simulink model "Klatt2"  (R2014a)
settings: Solver=ode45  StartTime=0  StopTime=6200  MaxStep=0.1  RelTol=1e-3
libraries: simulink x1
settings Model: Creator=OshoGupta  LastModifiedBy=abc
settings DataIOCC: SignalLoggingSaveFormat=ModelDataLogs
settings OptimizationCC: ExpressionDepthLimit=2147483647
settings DebuggingCC: UnderspecifiedInitializationDetection=Classic  FcnCallInpInsideContextMsg=EnableAllAsWarning  StateNameClashWarn=warning

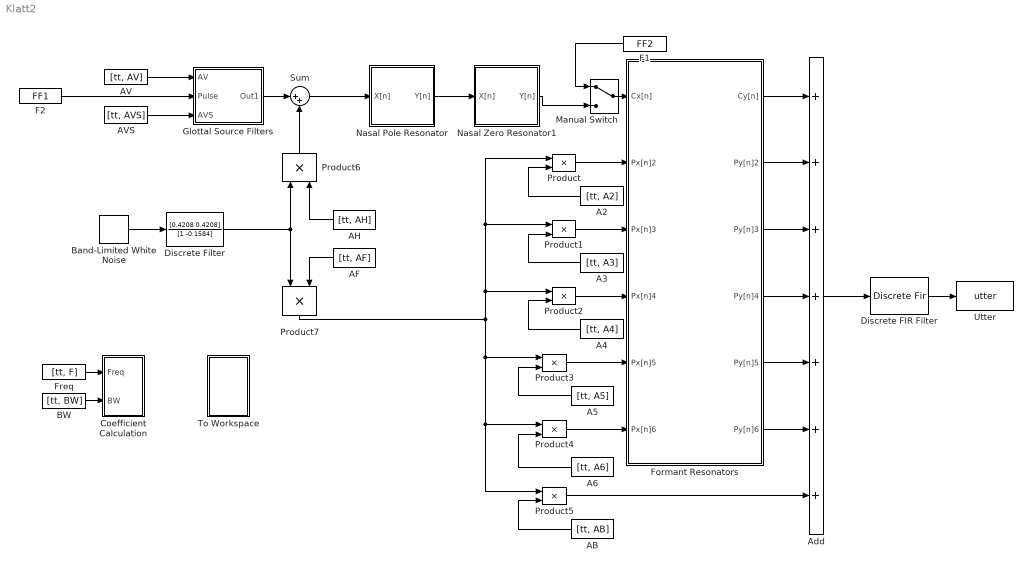
== system Klatt2 ==
  A2 : FromWorkspace  VariableName=[tt, A2]  SampleTime=0
  A3 : FromWorkspace  VariableName=[tt, A3]  SampleTime=0
  A4 : FromWorkspace  VariableName=[tt, A4]  SampleTime=0
  A5 : FromWorkspace  VariableName=[tt, A5]  SampleTime=0
  A6 : FromWorkspace  VariableName=[tt, A6]  SampleTime=0
  AB : FromWorkspace  VariableName=[tt, AB]  SampleTime=0
  AF : FromWorkspace  VariableName=[tt, AF]  SampleTime=0
  AH : FromWorkspace  VariableName=[tt, AH]  SampleTime=0
  AV : FromWorkspace  VariableName=[tt, AV]  SampleTime=0
  AVS : FromWorkspace  VariableName=[tt, AVS]  SampleTime=0
  Add : Sum  Inputs=+++++++
  BW : FromWorkspace  VariableName=[tt, BW]  SampleTime=0
  Band-Limited White Noise : simulink/Sources/Band-Limited White Noise  Cov=[0.1]  Ts=0.1  seed=[23341]
  Coefficient Calculation : Subsystem
  Discrete FIR Filter : DiscreteFir  Coefficients=[1 -0.98]
  Discrete Filter : DiscreteFilter  Numerator=[0.4208 0.4208]  Denominator=[1 -0.1584]
  F1 : FromWorkspace  VariableName=FF2  SampleTime=0
  F2 : FromWorkspace  VariableName=FF1  SampleTime=0
  Formant Resonators : Subsystem
  Freq : FromWorkspace  VariableName=[tt, F]  SampleTime=0
  Glottal Source Filters : Subsystem
  Manual Switch : ManualSwitch
  Nasal Pole Resonator : Subsystem
  Nasal Zero Resonator1 : Subsystem
  Product{,1..7} (8 alike) : Product  RndMeth=Zero
  Sum : Sum  Inputs=|++
  To Workspace : Subsystem
  Utter : ToWorkspace  VariableName=utter  SaveFormat=Timeseries  SampleTime=-1
  wires:
  Freq/1 -> Coefficient Calculation/1(Freq)
  BW/1 -> Coefficient Calculation/2(BW)
  Nasal Pole Resonator/1(Y[n]) -> Nasal Zero Resonator1/1(X[n])
  A2/1 -> Product/2
  Product/1 -> Formant Resonators/2(Px[n]2)
  A3/1 -> Product1/2
  Product1/1 -> Formant Resonators/3(Px[n]3)
  A4/1 -> Product2/2
  Product2/1 -> Formant Resonators/4(Px[n]4)
  A5/1 -> Product3/2
  Product3/1 -> Formant Resonators/5(Px[n]5)
  Product4/1 -> Formant Resonators/6(Px[n]6)
  AB/1 -> Product5/2
  Product7/1 -> Product4/1, Product5/1, Product3/1, Product/1, Product1/1, Product2/1
  Formant Resonators/1(Cy[n]) -> Add/1
  Formant Resonators/2(Py[n]2) -> Add/2
  Formant Resonators/3(Py[n]3) -> Add/3
  Formant Resonators/4(Py[n]4) -> Add/4
  Formant Resonators/5(Py[n]5) -> Add/5
  Formant Resonators/6(Py[n]6) -> Add/6
  Product5/1 -> Add/7
  A6/1 -> Product4/2
  Band-Limited White Noise/1 -> Discrete Filter/1
  Discrete Filter/1 -> Product7/1, Product6/1
  AH/1 -> Product6/2
  AF/1 -> Product7/2
  Sum/1 -> Nasal Pole Resonator/1(X[n])
  Nasal Zero Resonator1/1(Y[n]) -> Manual Switch/2
  F1/1 -> Manual Switch/1
  AVS/1 -> Glottal Source Filters/3(AVS)
  AV/1 -> Glottal Source Filters/1(AV)
  Glottal Source Filters/1(Out1) -> Sum/1
  Add/1 -> Discrete FIR Filter/1
  Discrete FIR Filter/1 -> Utter/1
  F2/1 -> Glottal Source Filters/2(Pulse)
  Manual Switch/1 -> Formant Resonators/1(Cx[n])
  Product6/1 -> Sum/2

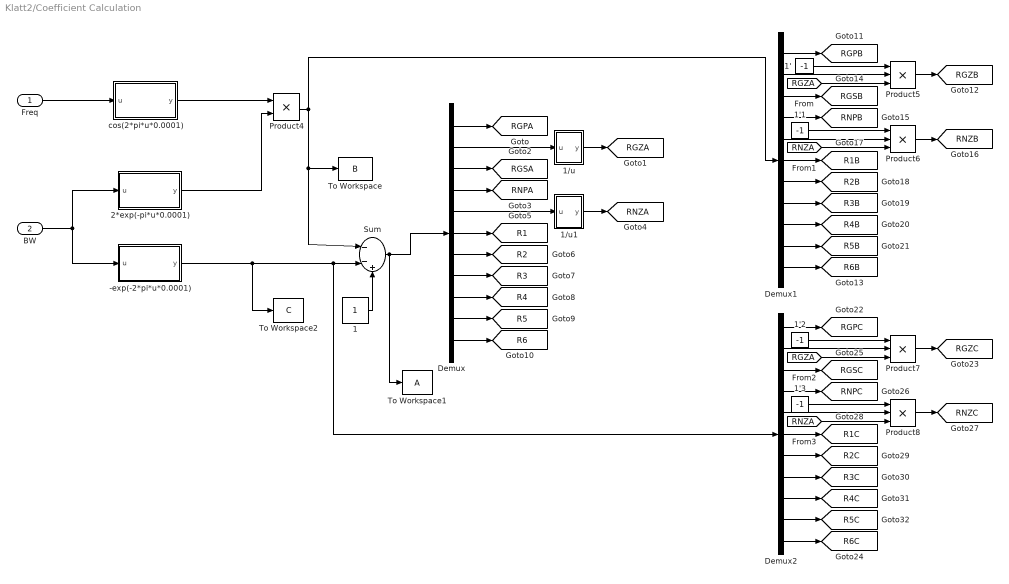
== system Klatt2/Coefficient Calculation ==
  Freq : Inport
  BW : Inport  Port=2
  -exp(-2*pi*u*0.0001) : MATLAB Function  TreatAsAtomicUnit=on
  1 : Constant
  1'{,1..3} (4 alike) : Constant  Value=-1
  1/u : MATLAB Function  TreatAsAtomicUnit=on
  1/u1 : MATLAB Function  TreatAsAtomicUnit=on
  2*exp(-pi*u*0.0001) : MATLAB Function  TreatAsAtomicUnit=on
  Demux : Demux  Outputs=11
  Demux1 : Demux  Outputs=11
  Demux2 : Demux  Outputs=11
  Product4 : Product  RndMeth=Zero
  Product5 : Product  Inputs=3  RndMeth=Zero
  Product6 : Product  Inputs=3  RndMeth=Zero
  Product7 : Product  Inputs=3  RndMeth=Zero
  Product8 : Product  Inputs=***  RndMeth=Zero
  Sum : Sum  Inputs=|--+
  To Workspace : ToWorkspace  VariableName=B  SaveFormat=Timeseries  SampleTime=-1
  To Workspace1 : ToWorkspace  VariableName=A  SaveFormat=Timeseries  SampleTime=-1
  To Workspace2 : ToWorkspace  VariableName=C  SaveFormat=Timeseries  SampleTime=-1
  cos(2*pi*u*0.0001) : MATLAB Function  TreatAsAtomicUnit=on
  tag scope: R1=global, R1B=global, R1C=global, R2=global, R2B=global, R2C=global, R3=global, R3B=global, R3C=global, R4=global, R4B=global, R4C=global, R5=global, R5B=global, R5C=global, R6=global, R6B=global, R6C=global, RGPA=global, RGPB=global, RGPC=global, RGSA=global, RGSB=global, RGSC=global, RGZA=global, RGZB=global, RGZC=global, RNPA=global, RNPB=global, RNPC=global, RNZA=global, RNZB=global, RNZC=global
  wires:
  BW/1 -> 2*exp(-pi*u*0.0001)/1(u), -exp(-2*pi*u*0.0001)/1(u)
  Freq/1 -> cos(2*pi*u*0.0001)/1(u)
  cos(2*pi*u*0.0001)/1(y) -> Product4/1
  2*exp(-pi*u*0.0001)/1(y) -> Product4/2
  Product4/1 -> Demux1/1, To Workspace/1, Sum/1
  -exp(-2*pi*u*0.0001)/1(y) -> To Workspace2/1, Sum/2, Demux2/1
  1/1 -> Sum/3
  Sum/1 -> Demux/1, To Workspace1/1
  Demux/1 -> [RGPA]
  Demux/3 -> [RGSA]
  Demux/4 -> [RNPA]
  Demux/6 -> [R1]
  Demux/7 -> [R2]
  Demux/8 -> [R3]
  Demux/9 -> [R4]
  Demux/10 -> [R5]
  Demux/11 -> [R6]
  Demux/5 -> 1/u1/1(u)
  1/u1/1(y) -> [RNZA]
  Product5/1 -> [RGZB]
  Demux1/2 -> Product5/2
  Demux1/1 -> [RGPB]
  Demux1/3 -> [RGSB]
  Demux1/4 -> [RNPB]
  Demux1/6 -> [R1B]
  Demux1/7 -> [R2B]
  Demux1/8 -> [R3B]
  Demux1/9 -> [R4B]
  Demux1/10 -> [R5B]
  Demux1/11 -> [R6B]
  Demux1/5 -> Product6/2
  Product6/1 -> [RNZB]
  1'/1 -> Product5/1
  [RGZA] -> Product5/3
  1'1/1 -> Product6/1
  [RNZA] -> Product6/3
  Product7/1 -> [RGZC]
  Demux2/2 -> Product7/2
  Demux2/1 -> [RGPC]
  Demux2/3 -> [RGSC]
  Demux2/4 -> [RNPC]
  Demux2/6 -> [R1C]
  Demux2/7 -> [R2C]
  Demux2/8 -> [R3C]
  Demux2/9 -> [R4C]
  Demux2/10 -> [R5C]
  Demux2/11 -> [R6C]
  Demux2/5 -> Product8/2
  Product8/1 -> [RNZC]
  1'2/1 -> Product7/1
  [RGZA] -> Product7/3
  1'3/1 -> Product8/1
  [RNZA] -> Product8/3
  Demux/2 -> 1/u/1(u)
  1/u/1(y) -> [RGZA]

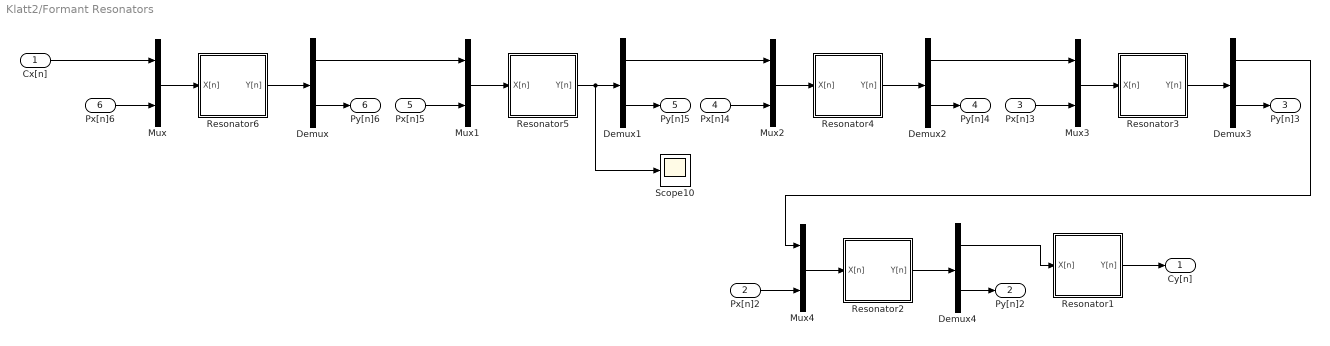
== system Klatt2/Formant Resonators ==
  Cx[n] : Inport
  Px[n]2 : Inport  Port=2
  Px[n]3 : Inport  Port=3
  Px[n]4 : Inport  Port=4
  Px[n]5 : Inport  Port=5
  Px[n]6 : Inport  Port=6
  Demux{,1..4} (5 alike) : Demux  Outputs=2
  Mux{,1..4} (5 alike) : Mux  Inputs=2
  Resonator1 : Subsystem
  Resonator2 : Subsystem
  Resonator3 : Subsystem
  Resonator4 : Subsystem
  Resonator5 : Subsystem
  Resonator6 : Subsystem
  Scope10 : Scope
  Cy[n] : Outport
  Py[n]2 : Outport  Port=2
  Py[n]3 : Outport  Port=3
  Py[n]4 : Outport  Port=4
  Py[n]5 : Outport  Port=5
  Py[n]6 : Outport  Port=6
  wires:
  Mux/1 -> Resonator6/1(X[n])
  Resonator6/1(Y[n]) -> Demux/1
  Demux/2 -> Py[n]6/1
  Cx[n]/1 -> Mux/1
  Px[n]6/1 -> Mux/2
  Mux1/1 -> Resonator5/1(X[n])
  Resonator5/1(Y[n]) -> Demux1/1, Scope10/1
  Demux1/2 -> Py[n]5/1
  Demux/1 -> Mux1/1
  Px[n]5/1 -> Mux1/2
  Mux2/1 -> Resonator4/1(X[n])
  Resonator4/1(Y[n]) -> Demux2/1
  Demux2/2 -> Py[n]4/1
  Demux1/1 -> Mux2/1
  Px[n]4/1 -> Mux2/2
  Mux3/1 -> Resonator3/1(X[n])
  Resonator3/1(Y[n]) -> Demux3/1
  Demux3/2 -> Py[n]3/1
  Demux2/1 -> Mux3/1
  Px[n]3/1 -> Mux3/2
  Mux4/1 -> Resonator2/1(X[n])
  Resonator2/1(Y[n]) -> Demux4/1
  Demux4/2 -> Py[n]2/1
  Demux3/1 -> Mux4/1
  Px[n]2/1 -> Mux4/2
  Resonator1/1(Y[n]) -> Cy[n]/1
  Demux4/1 -> Resonator1/1(X[n])

== system Klatt2/Glottal Source Filters ==
  note: Glottal Zero
      | Resonator
  note: Glottal Zero
      | Resonator
  AV : Inport
  Pulse : Inport  Port=2
  AVS : Inport  Port=3
  Glottal Pole Resonator : Subsystem
  Glottal Sinusoidal Resonator : Subsystem
  Nasal Zero Resonator1 : Subsystem
  Product : Product  RndMeth=Zero
  Product1 : Product  RndMeth=Zero
  Sum : Sum  Inputs=|++
  Out1 : Outport
  wires:
  Nasal Zero Resonator1/1(Y[n]) -> Product/2
  AV/1 -> Product/1
  Product/1 -> Sum/1
  Product1/1 -> Sum/2
  Glottal Pole Resonator/1(Y[n]) -> Glottal Sinusoidal Resonator/1(X[n]), Nasal Zero Resonator1/1(X[n])
  Sum/1 -> Out1/1
  Pulse/1 -> Glottal Pole Resonator/1(X[n])
  Glottal Sinusoidal Resonator/1(Y[n]) -> Product1/1
  AVS/1 -> Product1/2

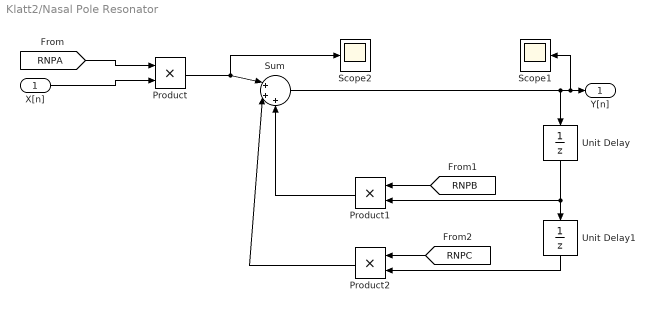
== system Klatt2/Nasal Pole Resonator ==
  X[n] : Inport
  Product : Product  RndMeth=Zero
  Product1 : Product  RndMeth=Zero
  Product2 : Product  RndMeth=Zero
  Scope1 : Scope
      settings: SaveName=ScopeData7
  Scope2 : Scope
      settings: SaveName=ScopeData6
  Sum : Sum  Inputs=|+++
  Unit Delay : UnitDelay  SampleTime=-1
  Unit Delay1 : UnitDelay  SampleTime=-1
  Y[n] : Outport
  wires:
  Product2/1 -> Sum/2
  Product1/1 -> Sum/3
  [RNPB] -> Product1/1
  Unit Delay1/1 -> Product2/2
  Unit Delay/1 -> Product1/2, Unit Delay1/1
  Sum/1 -> Y[n]/1, Scope1/1, Unit Delay/1
  Product/1 -> Sum/1, Scope2/1
  X[n]/1 -> Product/2
  [RNPA] -> Product/1
  [RNPC] -> Product2/1

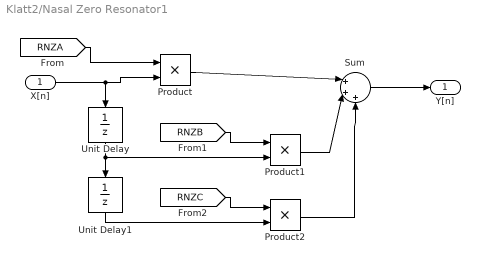
== system Klatt2/Nasal Zero Resonator1 ==
  X[n] : Inport
  Product : Product  RndMeth=Zero
  Product1 : Product  RndMeth=Zero
  Product2 : Product  RndMeth=Zero
  Sum : Sum  Inputs=|+++
  Unit Delay : UnitDelay  SampleTime=-1
  Unit Delay1 : UnitDelay  SampleTime=-1
  Y[n] : Outport
  wires:
  Product2/1 -> Sum/3
  Product1/1 -> Sum/2
  [RNZC] -> Product2/1
  [RNZB] -> Product1/1
  Unit Delay1/1 -> Product2/2
  Unit Delay/1 -> Product1/2, Unit Delay1/1
  Product/1 -> Sum/1
  X[n]/1 -> Product/2, Unit Delay/1
  [RNZA] -> Product/1
  Sum/1 -> Y[n]/1

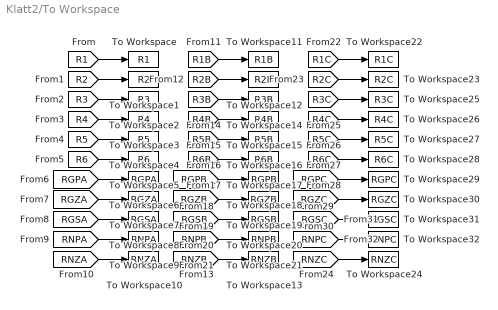
== system Klatt2/To Workspace ==
  To Workspace : ToWorkspace  VariableName=R1  SaveFormat=Timeseries  SampleTime=-1
  To Workspace1 : ToWorkspace  VariableName=R2  SaveFormat=Timeseries  SampleTime=-1
  To Workspace10 : ToWorkspace  VariableName=RNZA  SaveFormat=Timeseries  SampleTime=-1
  To Workspace11 : ToWorkspace  VariableName=R1B  SaveFormat=Timeseries  SampleTime=-1
  To Workspace12 : ToWorkspace  VariableName=R2B  SaveFormat=Timeseries  SampleTime=-1
  To Workspace13 : ToWorkspace  VariableName=RNZB  SaveFormat=Timeseries  SampleTime=-1
  To Workspace14 : ToWorkspace  VariableName=R3B  SaveFormat=Timeseries  SampleTime=-1
  To Workspace15 : ToWorkspace  VariableName=R4B  SaveFormat=Timeseries  SampleTime=-1
  To Workspace16 : ToWorkspace  VariableName=R5B  SaveFormat=Timeseries  SampleTime=-1
  To Workspace17 : ToWorkspace  VariableName=R6B  SaveFormat=Timeseries  SampleTime=-1
  To Workspace18 : ToWorkspace  VariableName=RGPB  SaveFormat=Timeseries  SampleTime=-1
  To Workspace19 : ToWorkspace  VariableName=RGZB  SaveFormat=Timeseries  SampleTime=-1
  To Workspace2 : ToWorkspace  VariableName=R3  SaveFormat=Timeseries  SampleTime=-1
  To Workspace20 : ToWorkspace  VariableName=RGSB  SaveFormat=Timeseries  SampleTime=-1
  To Workspace21 : ToWorkspace  VariableName=RNPB  SaveFormat=Timeseries  SampleTime=-1
  To Workspace22 : ToWorkspace  VariableName=R1C  SaveFormat=Timeseries  SampleTime=-1
  To Workspace23 : ToWorkspace  VariableName=R2C  SaveFormat=Timeseries  SampleTime=-1
  To Workspace24 : ToWorkspace  VariableName=RNZC  SaveFormat=Timeseries  SampleTime=-1
  To Workspace25 : ToWorkspace  VariableName=R3C  SaveFormat=Timeseries  SampleTime=-1
  To Workspace26 : ToWorkspace  VariableName=R4C  SaveFormat=Timeseries  SampleTime=-1
  To Workspace27 : ToWorkspace  VariableName=R5C  SaveFormat=Timeseries  SampleTime=-1
  To Workspace28 : ToWorkspace  VariableName=R6C  SaveFormat=Timeseries  SampleTime=-1
  To Workspace29 : ToWorkspace  VariableName=RGPC  SaveFormat=Timeseries  SampleTime=-1
  To Workspace3 : ToWorkspace  VariableName=R4  SaveFormat=Timeseries  SampleTime=-1
  To Workspace30 : ToWorkspace  VariableName=RGZC  SaveFormat=Timeseries  SampleTime=-1
  To Workspace31 : ToWorkspace  VariableName=RGSC  SaveFormat=Timeseries  SampleTime=-1
  To Workspace32 : ToWorkspace  VariableName=RNPC  SaveFormat=Timeseries  SampleTime=-1
  To Workspace4 : ToWorkspace  VariableName=R5  SaveFormat=Timeseries  SampleTime=-1
  To Workspace5 : ToWorkspace  VariableName=R6  SaveFormat=Timeseries  SampleTime=-1
  To Workspace6 : ToWorkspace  VariableName=RGPA  SaveFormat=Timeseries  SampleTime=-1
  To Workspace7 : ToWorkspace  VariableName=RGZA  SaveFormat=Timeseries  SampleTime=-1
  To Workspace8 : ToWorkspace  VariableName=RGSA  SaveFormat=Timeseries  SampleTime=-1
  To Workspace9 : ToWorkspace  VariableName=RNPA  SaveFormat=Timeseries  SampleTime=-1
  wires:
  [R1] -> To Workspace/1
  [R2] -> To Workspace1/1
  [R3] -> To Workspace2/1
  [R4] -> To Workspace3/1
  [R5] -> To Workspace4/1
  [R6] -> To Workspace5/1
  [RGPA] -> To Workspace6/1
  [RGZA] -> To Workspace7/1
  [RGSA] -> To Workspace8/1
  [RNPA] -> To Workspace9/1
  [RNZA] -> To Workspace10/1
  [R1B] -> To Workspace11/1
  [R2B] -> To Workspace12/1
  [R3B] -> To Workspace14/1
  [R4B] -> To Workspace15/1
  [R5B] -> To Workspace16/1
  [R6B] -> To Workspace17/1
  [RGPB] -> To Workspace18/1
  [RGZB] -> To Workspace19/1
  [RGSB] -> To Workspace20/1
  [RNPB] -> To Workspace21/1
  [RNZB] -> To Workspace13/1
  [R1C] -> To Workspace22/1
  [R2C] -> To Workspace23/1
  [R3C] -> To Workspace25/1
  [R4C] -> To Workspace26/1
  [R5C] -> To Workspace27/1
  [R6C] -> To Workspace28/1
  [RGPC] -> To Workspace29/1
  [RGZC] -> To Workspace30/1
  [RGSC] -> To Workspace31/1
  [RNPC] -> To Workspace32/1
  [RNZC] -> To Workspace24/1

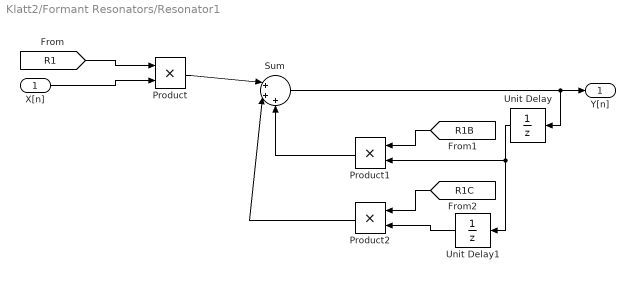
== system Klatt2/Formant Resonators/Resonator1 ==
  X[n] : Inport
  Product : Product  RndMeth=Zero
  Product1 : Product  RndMeth=Zero
  Product2 : Product  RndMeth=Zero
  Sum : Sum  Inputs=|+++
  Unit Delay : UnitDelay  SampleTime=-1
  Unit Delay1 : UnitDelay  SampleTime=-1
  Y[n] : Outport
  wires:
  Product2/1 -> Sum/2
  Product1/1 -> Sum/3
  [R1C] -> Product2/1
  [R1B] -> Product1/1
  Unit Delay1/1 -> Product2/2
  Unit Delay/1 -> Product1/2, Unit Delay1/1
  Sum/1 -> Y[n]/1, Unit Delay/1
  Product/1 -> Sum/1
  X[n]/1 -> Product/2
  [R1] -> Product/1

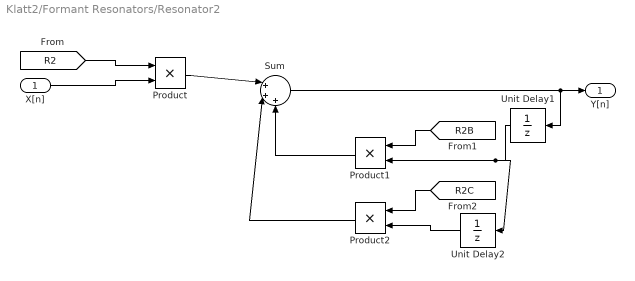
== system Klatt2/Formant Resonators/Resonator2 ==
  X[n] : Inport
  Product : Product  RndMeth=Zero
  Product1 : Product  RndMeth=Zero
  Product2 : Product  RndMeth=Zero
  Sum : Sum  Inputs=|+++
  Unit Delay1 : UnitDelay  SampleTime=-1
  Unit Delay2 : UnitDelay  SampleTime=-1
  Y[n] : Outport
  wires:
  Product2/1 -> Sum/2
  Product1/1 -> Sum/3
  [R2C] -> Product2/1
  [R2B] -> Product1/1
  Unit Delay2/1 -> Product2/2
  Unit Delay1/1 -> Product1/2, Unit Delay2/1
  Sum/1 -> Y[n]/1, Unit Delay1/1
  Product/1 -> Sum/1
  X[n]/1 -> Product/2
  [R2] -> Product/1

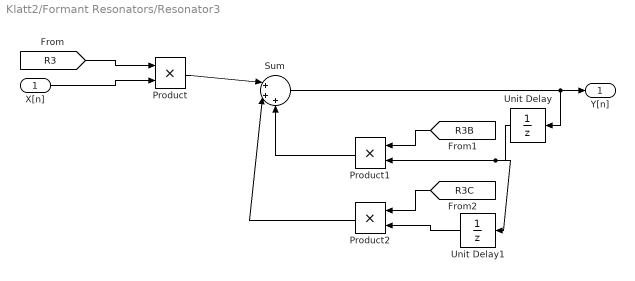
== system Klatt2/Formant Resonators/Resonator3 ==
  X[n] : Inport
  Product : Product  RndMeth=Zero
  Product1 : Product  RndMeth=Zero
  Product2 : Product  RndMeth=Zero
  Sum : Sum  Inputs=|+++
  Unit Delay : UnitDelay  SampleTime=-1
  Unit Delay1 : UnitDelay  SampleTime=-1
  Y[n] : Outport
  wires:
  Product2/1 -> Sum/2
  Product1/1 -> Sum/3
  [R3C] -> Product2/1
  [R3B] -> Product1/1
  Unit Delay1/1 -> Product2/2
  Unit Delay/1 -> Product1/2, Unit Delay1/1
  Sum/1 -> Y[n]/1, Unit Delay/1
  Product/1 -> Sum/1
  X[n]/1 -> Product/2
  [R3] -> Product/1

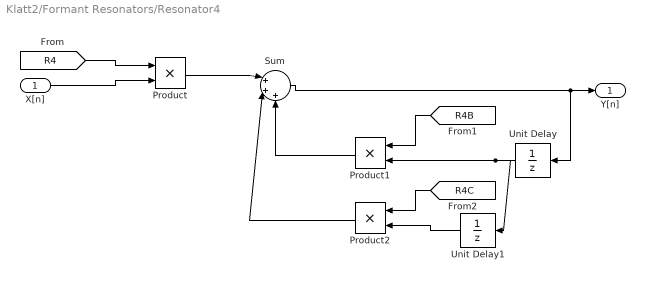
== system Klatt2/Formant Resonators/Resonator4 ==
  X[n] : Inport
  Product : Product  RndMeth=Zero
  Product1 : Product  RndMeth=Zero
  Product2 : Product  RndMeth=Zero
  Sum : Sum  Inputs=|+++
  Unit Delay : UnitDelay  SampleTime=-1
  Unit Delay1 : UnitDelay  SampleTime=-1
  Y[n] : Outport
  wires:
  Product2/1 -> Sum/2
  Product1/1 -> Sum/3
  [R4C] -> Product2/1
  [R4B] -> Product1/1
  Unit Delay1/1 -> Product2/2
  Unit Delay/1 -> Product1/2, Unit Delay1/1
  Sum/1 -> Y[n]/1, Unit Delay/1
  Product/1 -> Sum/1
  X[n]/1 -> Product/2
  [R4] -> Product/1

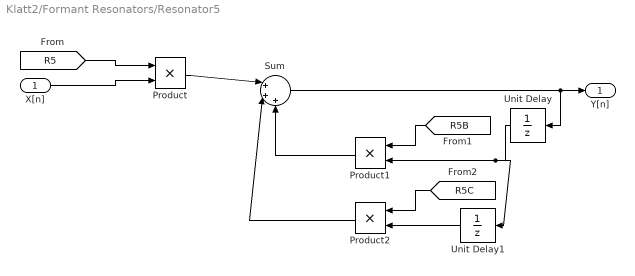
== system Klatt2/Formant Resonators/Resonator5 ==
  X[n] : Inport
  Product : Product  RndMeth=Zero
  Product1 : Product  RndMeth=Zero
  Product2 : Product  RndMeth=Zero
  Sum : Sum  Inputs=|+++
  Unit Delay : UnitDelay  SampleTime=-1
  Unit Delay1 : UnitDelay  SampleTime=-1
  Y[n] : Outport
  wires:
  Product2/1 -> Sum/2
  Product1/1 -> Sum/3
  [R5C] -> Product2/1
  [R5B] -> Product1/1
  Unit Delay1/1 -> Product2/2
  Unit Delay/1 -> Product1/2, Unit Delay1/1
  Sum/1 -> Y[n]/1, Unit Delay/1
  Product/1 -> Sum/1
  X[n]/1 -> Product/2
  [R5] -> Product/1

== system Klatt2/Formant Resonators/Resonator6 ==
  X[n] : Inport
  Product : Product  RndMeth=Zero
  Product1 : Product  RndMeth=Zero
  Product2 : Product  RndMeth=Zero
  Sum : Sum  Inputs=|+++
  Unit Delay : UnitDelay  SampleTime=-1
  Unit Delay1 : UnitDelay  SampleTime=-1
  Y[n] : Outport
  wires:
  Product2/1 -> Sum/2
  Product1/1 -> Sum/3
  [R6C] -> Product2/1
  [R6B] -> Product1/1
  Unit Delay1/1 -> Product2/2
  Unit Delay/1 -> Product1/2, Unit Delay1/1
  Sum/1 -> Y[n]/1, Unit Delay/1
  Product/1 -> Sum/1
  X[n]/1 -> Product/2
  [R6] -> Product/1

== system Klatt2/Glottal Source Filters/Glottal Pole Resonator ==
  X[n] : Inport
  Product : Product  RndMeth=Zero
  Product1 : Product  RndMeth=Zero
  Product2 : Product  RndMeth=Zero
  Sum : Sum  Inputs=|+++
  Unit Delay1 : UnitDelay  SampleTime=-1
  Unit Delay2 : UnitDelay  SampleTime=-1
  Y[n] : Outport
  wires:
  Product2/1 -> Sum/2
  Product1/1 -> Sum/3
  [RGPC] -> Product2/1
  [RGPB] -> Product1/1
  Unit Delay1/1 -> Product2/2
  Unit Delay2/1 -> Product1/2, Unit Delay1/1
  Sum/1 -> Y[n]/1, Unit Delay2/1
  Product/1 -> Sum/1
  X[n]/1 -> Product/2
  [RGPA] -> Product/1

== system Klatt2/Glottal Source Filters/Glottal Sinusoidal Resonator ==
  X[n] : Inport
  Product : Product  RndMeth=Zero
  Product1 : Product  RndMeth=Zero
  Product2 : Product  RndMeth=Zero
  Sum : Sum  Inputs=|+++
  Unit Delay1 : UnitDelay  SampleTime=-1
  Unit Delay2 : UnitDelay  SampleTime=-1
  Y[n] : Outport
  wires:
  [RGSA] -> Product/1
  X[n]/1 -> Product/2
  Product/1 -> Sum/1
  Sum/1 -> Y[n]/1, Unit Delay2/1
  Unit Delay2/1 -> Product1/2, Unit Delay1/1
  Unit Delay1/1 -> Product2/2
  [RGSB] -> Product1/1
  [RGSC] -> Product2/1
  Product1/1 -> Sum/3
  Product2/1 -> Sum/2

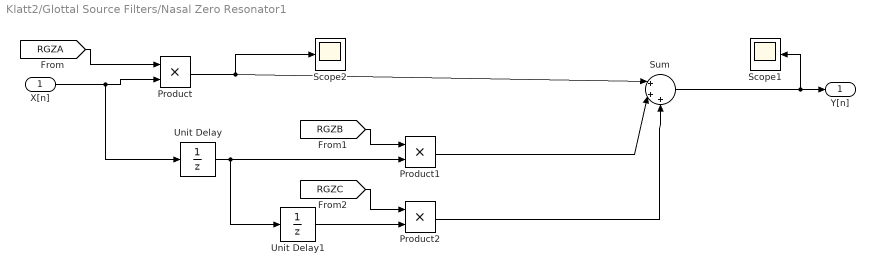
== system Klatt2/Glottal Source Filters/Nasal Zero Resonator1 ==
  X[n] : Inport
  Product : Product  RndMeth=Zero
  Product1 : Product  RndMeth=Zero
  Product2 : Product  RndMeth=Zero
  Scope1 : Scope
      settings: SaveName=ScopeData7
  Scope2 : Scope
      settings: SaveName=ScopeData6
  Sum : Sum  Inputs=|+++
  Unit Delay : UnitDelay  SampleTime=-1
  Unit Delay1 : UnitDelay  SampleTime=-1
  Y[n] : Outport
  wires:
  Product2/1 -> Sum/3
  Product1/1 -> Sum/2
  [RGZC] -> Product2/1
  [RGZB] -> Product1/1
  Unit Delay1/1 -> Product2/2
  Unit Delay/1 -> Product1/2, Unit Delay1/1
  Product/1 -> Sum/1, Scope2/1
  X[n]/1 -> Product/2, Unit Delay/1
  [RGZA] -> Product/1
  Sum/1 -> Y[n]/1, Scope1/1

== matlab function Klatt2/Coefficient Calculation/1//u1 ==
  data: u input; y output
function y = fcn(u)
%#codegen
y = 1/u;

== matlab function Klatt2/Coefficient Calculation/2*exp(-pi*u*0.0001) ==
  data: u input; y output
function y = fcn(u)
%#codegen
y = 2*exp(-pi*u*0.0001);

== matlab function Klatt2/Coefficient Calculation/cos(2*pi*u*0.0001) ==
  data: u input; y output
function y = fcn(u)
%#codegen
y = cos(2*pi*u*0.0001);

== matlab function Klatt2/Coefficient Calculation/1//u ==
  data: u input; y output
function y = fcn(u)
%#codegen
y = 1/u;

== matlab function Klatt2/Coefficient Calculation/-exp(-2*pi*u*0.0001) ==
  data: u input; y output
function y = fcn(u)
%#codegen
y = -exp(-2*pi*u*0.0001);
